simulink model "SimpleEKF_2007a"  (Simulink 6.6)
settings: Solver=FixedStepDiscrete  StartTime=0.0  StopTime=300  FixedStep=0.01  RelTol=1e-3
values from neighbouring files (symbols this model uses):
  initP = diag([ 1 1 1 1e5 1e5 1 1e5 1e5 1e5 ])    [SimpleEKF_init.m.m]
undefined symbols (not defined in the file or in its folder): DiscIntNeverNeededParam, gcbh, hwbcalib_subsystem
libraries: simulink x8, dspmtrx3 x5, dspinverses x1
(part 5 of 9)

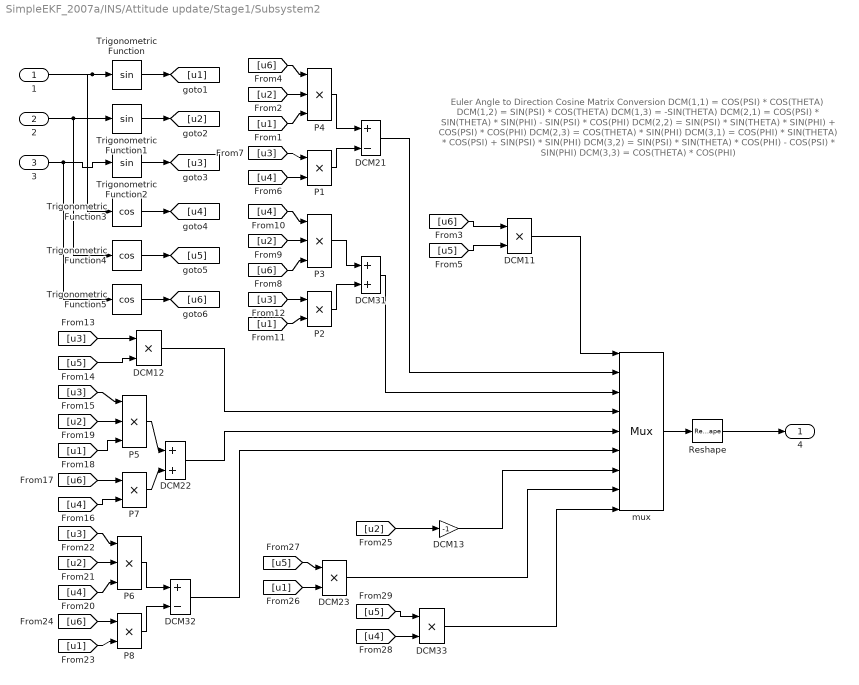
== system SimpleEKF_2007a/INS/Attitude update/Stage1/Subsystem2 ==
  note: Euler Angle to Direction Cosine Matrix Conversion
      |
      | DCM(1,1) = COS(PSI) * COS(THETA)
      | DCM(1,2) = SIN(PSI) * COS(THETA)
      | DCM(1,3) = -SIN(THETA)
      | DCM(2,1) = COS(PSI) * SIN(THETA) * SIN(PHI) - SIN(PSI) * COS(PHI)
      | DCM(2,2) = SIN(PSI) * SIN(THETA) * SIN(PHI) + COS(PSI) * COS(PHI)
      | DCM(2,3) = COS(THETA) * SIN(PHI)
      | DCM(3,1) = COS(PHI) * SIN(THETA) * COS(PSI) + SIN(PSI) * SIN(PHI)
      | DCM(3,2) = SIN(PSI) * SIN(THETA) * COS(PHI) - COS(PSI) * SIN(PHI)
      | DCM(3,3) = COS(THETA) * COS(PHI)
  1 : Inport  PortDimensions=1  DataType=double  OutDataType=fixdt(1,16,0)  OutScaling=[]
  2 : Inport  Port=2  PortDimensions=1  DataType=double  OutDataType=fixdt(1,16,0)  OutScaling=[]
  3 : Inport  Port=3  PortDimensions=1  DataType=double  OutDataType=fixdt(1,16,0)  OutScaling=[]
  DCM11 : Product  Tag=MBDLibrary v2007b.1  OutDataType=fixdt(1,16,0)  OutScaling=[]  RndMeth=Zero  InputSameDT=on  mask(Product (MBDLibrary)){Inputs_mbdlib=2}
      mask prompts: Inputs_mbdlib "Number of Inputs"
      mask help: Multiplies inputs.
      settings: OpenFcn=|
      | if exist('mbdlib_dialog')
      |    mbdlib_dialog(gcb,'open')
      | else
      |    open_system(gcb, 'mask')
      | end
      mask Help: The PRODUCT block is used to multiply inputs.
  DCM12 : Product  Tag=MBDLibrary v2007b.1  OutDataType=fixdt(1,16,0)  OutScaling=[]  RndMeth=Zero  InputSameDT=on  mask(Product (MBDLibrary)){Inputs_mbdlib=2}
      mask prompts: Inputs_mbdlib "Number of Inputs"
      mask help: Multiplies inputs.
      settings: OpenFcn=|
      | if exist('mbdlib_dialog')
      |    mbdlib_dialog(gcb,'open')
      | else
      |    open_system(gcb, 'mask')
      | end
      mask Help: The PRODUCT block is used to multiply inputs.
  DCM13 : Gain  Tag=MBDLibrary v2007b.1  Gain=-1  ParameterDataType=fixdt(1,16,0)  ParameterScaling=[]  OutDataType=fixdt(1,16,0)  OutScaling=[]  RndMeth=Zero  mask(Gain (MBDLibrary)){gain_mbdlib=-1}
      mask prompts: gain_mbdlib "Gain"
      mask help: Multiplies the input by the gain.
      settings: OpenFcn=|
      | if exist('mbdlib_dialog')
      |    mbdlib_dialog(gcb,'open')
      | else
      |    open_system(gcb, 'mask')
      | end
      mask Help: The GAIN block multiplies the input by the gain value.  This block may accept any data types other than boolean.  The user must take care to not use a non-integer gain for int32/uint32 inputs.
      mask Display: disp([get_param(gcb, 'Gain') 'x'])
  DCM21 : Sum  Tag=MBDLibrary v2007b.1  Inputs=+-  OutDataType=fixdt(1,16,0)  OutScaling=[]  RndMeth=Zero  InputSameDT=on  mask(Sum (MBDLibrary)){inputs_mbdlib=+-}
      mask prompts: inputs_mbdlib "List of signs"
      mask help: Adds values together.
      settings: OpenFcn=|
      | if exist('mbdlib_dialog')
      |    mbdlib_dialog(gcb,'open')
      | else
      |    open_system(gcb, 'mask')
      | end
      mask Help:
      | The SUM block is used to add or subtract  inputs.
      | The inputs may be specified as:
      |   (a) + or - for each port (i.e. ++-+)
      |   (b) An integer to indicate the number of ports to add
      | Note that the number of ports input to this block must be between 1 and 25.
      | When only 1 inport is selected, the block computes the summation of vector input elements and outputs a scalar.
  DCM22 : Sum  Tag=MBDLibrary v2007b.1  OutDataType=fixdt(1,16,0)  OutScaling=[]  RndMeth=Zero  InputSameDT=on  mask(Sum (MBDLibrary)){inputs_mbdlib=++}
      mask prompts: inputs_mbdlib "List of signs"
      mask help: Adds values together.
      settings: OpenFcn=|
      | if exist('mbdlib_dialog')
      |    mbdlib_dialog(gcb,'open')
      | else
      |    open_system(gcb, 'mask')
      | end
      mask Help:
      | The SUM block is used to add or subtract  inputs.
      | The inputs may be specified as:
      |   (a) + or - for each port (i.e. ++-+)
      |   (b) An integer to indicate the number of ports to add
      | Note that the number of ports input to this block must be between 1 and 25.
      | When only 1 inport is selected, the block computes the summation of vector input elements and outputs a scalar.
  DCM23 : Product  Tag=MBDLibrary v2007b.1  OutDataType=fixdt(1,16,0)  OutScaling=[]  RndMeth=Zero  InputSameDT=on  mask(Product (MBDLibrary)){Inputs_mbdlib=2}
      mask prompts: Inputs_mbdlib "Number of Inputs"
      mask help: Multiplies inputs.
      settings: OpenFcn=|
      | if exist('mbdlib_dialog')
      |    mbdlib_dialog(gcb,'open')
      | else
      |    open_system(gcb, 'mask')
      | end
      mask Help: The PRODUCT block is used to multiply inputs.
  DCM31 : Sum  Tag=MBDLibrary v2007b.1  OutDataType=fixdt(1,16,0)  OutScaling=[]  RndMeth=Zero  InputSameDT=on  mask(Sum (MBDLibrary)){inputs_mbdlib=++}
      mask prompts: inputs_mbdlib "List of signs"
      mask help: Adds values together.
      settings: OpenFcn=|
      | if exist('mbdlib_dialog')
      |    mbdlib_dialog(gcb,'open')
      | else
      |    open_system(gcb, 'mask')
      | end
      mask Help:
      | The SUM block is used to add or subtract  inputs.
      | The inputs may be specified as:
      |   (a) + or - for each port (i.e. ++-+)
      |   (b) An integer to indicate the number of ports to add
      | Note that the number of ports input to this block must be between 1 and 25.
      | When only 1 inport is selected, the block computes the summation of vector input elements and outputs a scalar.
  DCM32 : Sum  Tag=MBDLibrary v2007b.1  Inputs=+-  OutDataType=fixdt(1,16,0)  OutScaling=[]  RndMeth=Zero  InputSameDT=on  mask(Sum (MBDLibrary)){inputs_mbdlib=+-}
      mask prompts: inputs_mbdlib "List of signs"
      mask help: Adds values together.
      settings: OpenFcn=|
      | if exist('mbdlib_dialog')
      |    mbdlib_dialog(gcb,'open')
      | else
      |    open_system(gcb, 'mask')
      | end
      mask Help:
      | The SUM block is used to add or subtract  inputs.
      | The inputs may be specified as:
      |   (a) + or - for each port (i.e. ++-+)
      |   (b) An integer to indicate the number of ports to add
      | Note that the number of ports input to this block must be between 1 and 25.
      | When only 1 inport is selected, the block computes the summation of vector input elements and outputs a scalar.
  DCM33 : Product  Tag=MBDLibrary v2007b.1  OutDataType=fixdt(1,16,0)  OutScaling=[]  RndMeth=Zero  InputSameDT=on  mask(Product (MBDLibrary)){Inputs_mbdlib=2}
      mask prompts: Inputs_mbdlib "Number of Inputs"
      mask help: Multiplies inputs.
      settings: OpenFcn=|
      | if exist('mbdlib_dialog')
      |    mbdlib_dialog(gcb,'open')
      | else
      |    open_system(gcb, 'mask')
      | end
      mask Help: The PRODUCT block is used to multiply inputs.
  P1 : Product  Tag=MBDLibrary v2007b.1  OutDataType=fixdt(1,16,0)  OutScaling=[]  RndMeth=Zero  InputSameDT=on  mask(Product (MBDLibrary)){Inputs_mbdlib=2}
      mask prompts: Inputs_mbdlib "Number of Inputs"
      mask help: Multiplies inputs.
      settings: OpenFcn=|
      | if exist('mbdlib_dialog')
      |    mbdlib_dialog(gcb,'open')
      | else
      |    open_system(gcb, 'mask')
      | end
      mask Help: The PRODUCT block is used to multiply inputs.
  P2 : Product  Tag=MBDLibrary v2007b.1  OutDataType=fixdt(1,16,0)  OutScaling=[]  RndMeth=Zero  InputSameDT=on  mask(Product (MBDLibrary)){Inputs_mbdlib=2}
      mask prompts: Inputs_mbdlib "Number of Inputs"
      mask help: Multiplies inputs.
      settings: OpenFcn=|
      | if exist('mbdlib_dialog')
      |    mbdlib_dialog(gcb,'open')
      | else
      |    open_system(gcb, 'mask')
      | end
      mask Help: The PRODUCT block is used to multiply inputs.
  P3 : Product  Tag=MBDLibrary v2007b.1  Inputs=3  OutDataType=fixdt(1,16,0)  OutScaling=[]  RndMeth=Zero  InputSameDT=on  mask(Product (MBDLibrary)){Inputs_mbdlib=3}
      mask prompts: Inputs_mbdlib "Number of Inputs"
      mask help: Multiplies inputs.
      settings: OpenFcn=|
      | if exist('mbdlib_dialog')
      |    mbdlib_dialog(gcb,'open')
      | else
      |    open_system(gcb, 'mask')
      | end
      mask Help: The PRODUCT block is used to multiply inputs.
  P4 : Product  Tag=MBDLibrary v2007b.1  Inputs=3  OutDataType=fixdt(1,16,0)  OutScaling=[]  RndMeth=Zero  InputSameDT=on  mask(Product (MBDLibrary)){Inputs_mbdlib=3}
      mask prompts: Inputs_mbdlib "Number of Inputs"
      mask help: Multiplies inputs.
      settings: OpenFcn=|
      | if exist('mbdlib_dialog')
      |    mbdlib_dialog(gcb,'open')
      | else
      |    open_system(gcb, 'mask')
      | end
      mask Help: The PRODUCT block is used to multiply inputs.
  P5 : Product  Tag=MBDLibrary v2007b.1  Inputs=3  OutDataType=fixdt(1,16,0)  OutScaling=[]  RndMeth=Zero  InputSameDT=on  mask(Product (MBDLibrary)){Inputs_mbdlib=3}
      mask prompts: Inputs_mbdlib "Number of Inputs"
      mask help: Multiplies inputs.
      settings: OpenFcn=|
      | if exist('mbdlib_dialog')
      |    mbdlib_dialog(gcb,'open')
      | else
      |    open_system(gcb, 'mask')
      | end
      mask Help: The PRODUCT block is used to multiply inputs.
  P6 : Product  Tag=MBDLibrary v2007b.1  Inputs=3  OutDataType=fixdt(1,16,0)  OutScaling=[]  RndMeth=Zero  InputSameDT=on  mask(Product (MBDLibrary)){Inputs_mbdlib=3}
      mask prompts: Inputs_mbdlib "Number of Inputs"
      mask help: Multiplies inputs.
      settings: OpenFcn=|
      | if exist('mbdlib_dialog')
      |    mbdlib_dialog(gcb,'open')
      | else
      |    open_system(gcb, 'mask')
      | end
      mask Help: The PRODUCT block is used to multiply inputs.
  P7 : Product  Tag=MBDLibrary v2007b.1  OutDataType=fixdt(1,16,0)  OutScaling=[]  RndMeth=Zero  InputSameDT=on  mask(Product (MBDLibrary)){Inputs_mbdlib=2}
      mask prompts: Inputs_mbdlib "Number of Inputs"
      mask help: Multiplies inputs.
      settings: OpenFcn=|
      | if exist('mbdlib_dialog')
      |    mbdlib_dialog(gcb,'open')
      | else
      |    open_system(gcb, 'mask')
      | end
      mask Help: The PRODUCT block is used to multiply inputs.
  P8 : Product  Tag=MBDLibrary v2007b.1  OutDataType=fixdt(1,16,0)  OutScaling=[]  RndMeth=Zero  InputSameDT=on  mask(Product (MBDLibrary)){Inputs_mbdlib=2}
      mask prompts: Inputs_mbdlib "Number of Inputs"
      mask help: Multiplies inputs.
      settings: OpenFcn=|
      | if exist('mbdlib_dialog')
      |    mbdlib_dialog(gcb,'open')
      | else
      |    open_system(gcb, 'mask')
      | end
      mask Help: The PRODUCT block is used to multiply inputs.
  Reshape : Reshape  OutputDimensionality=Customize  OutputDimensions=[3,3]
  Trigonometric Function : Trigonometry
  Trigonometric Function1 : Trigonometry
  Trigonometric Function2 : Trigonometry
  Trigonometric Function3 : Trigonometry  Operator=cos
  Trigonometric Function4 : Trigonometry  Operator=cos
  Trigonometric Function5 : Trigonometry  Operator=cos
  mux : Mux  Tag=MBDLibrary v2007b.1  Inputs=9  mask(Mux (MBDLibrary)){Inputs_mbdlib=9}
      mask prompts: Inputs_mbdlib "Number of Inputs"
      mask help: Converts multipule inputs to a vector.
      settings: OpenFcn=|
      | if exist('mbdlib_dialog')
      |    mbdlib_dialog(gcb,'open')
      | else
      |    open_system(gcb, 'mask')
      | end
      mask Help: The MUX block provides a vector output to the model for separate inputs.  The output order will correspond to the input order (from the first input at the top of the block to the last input at the bottom of the block).
  4 : Outport  OutDataType=fixdt(1,16,0)  OutScaling=[]  InitialOutput=0
  wires:
  [u6] -> P3/3
  [u2] -> P3/2
  [u4] -> P3/1
  mux/1 -> Reshape/1
  DCM12/1 -> mux/4
  Reshape/1 -> 4/1
  1/1 -> Trigonometric Function/1, Trigonometric Function3/1
  2/1 -> Trigonometric Function1/1, Trigonometric Function4/1
  3/1 -> Trigonometric Function2/1, Trigonometric Function5/1
  Trigonometric Function/1 -> [u1]
  Trigonometric Function1/1 -> [u2]
  Trigonometric Function2/1 -> [u3]
  Trigonometric Function3/1 -> [u4]
  Trigonometric Function4/1 -> [u5]
  Trigonometric Function5/1 -> [u6]
  [u6] -> P4/1
  [u2] -> P4/2
  [u1] -> P4/3
  [u3] -> P1/1
  [u4] -> P1/2
  P4/1 -> DCM21/1
  P1/1 -> DCM21/2
  [u3] -> P2/1
  [u1] -> P2/2
  P3/1 -> DCM31/1
  P2/1 -> DCM31/2
  DCM21/1 -> mux/2
  DCM31/1 -> mux/3
  [u3] -> DCM12/1
  [u5] -> DCM12/2
  [u3] -> P5/1
  [u2] -> P5/2
  [u1] -> P5/3
  [u6] -> P7/1
  [u4] -> P7/2
  P5/1 -> DCM22/1
  P7/1 -> DCM22/2
  DCM22/1 -> mux/5
  [u3] -> P6/1
  [u2] -> P6/2
  [u4] -> P6/3
  [u6] -> P8/1
  [u1] -> P8/2
  P6/1 -> DCM32/1
  P8/1 -> DCM32/2
  DCM32/1 -> mux/6
  [u6] -> DCM11/1
  [u5] -> DCM11/2
  DCM11/1 -> mux/1
  [u2] -> DCM13/1
  DCM13/1 -> mux/7
  [u1] -> DCM23/2
  [u5] -> DCM23/1
  DCM23/1 -> mux/8
  [u4] -> DCM33/2
  [u5] -> DCM33/1
  DCM33/1 -> mux/9

== system SimpleEKF_2007a/INS/Attitude update/Stage1/square ==
  squareLibIn : Inport  DataType=double  OutDataType=fixdt(1,16,0)  OutScaling=[]
  Product : Product  OutDataType=fixdt(1,16,0)  OutScaling=[]  RndMeth=Zero
  squareLibOut : Outport  OutDataType=fixdt(1,16,0)  OutScaling=[]  InitialOutput=0
  wires:
  squareLibIn/1 -> Product/2, Product/1
  Product/1 -> squareLibOut/1

== system SimpleEKF_2007a/INS/Attitude update/Stage1/square1 ==
  squareLibIn : Inport  DataType=double  OutDataType=fixdt(1,16,0)  OutScaling=[]
  Product : Product  OutDataType=fixdt(1,16,0)  OutScaling=[]  RndMeth=Zero
  squareLibOut : Outport  OutDataType=fixdt(1,16,0)  OutScaling=[]  InitialOutput=0
  wires:
  squareLibIn/1 -> Product/2, Product/1
  Product/1 -> squareLibOut/1

== system SimpleEKF_2007a/INS/Attitude update/Stage1/square2 ==
  squareLibIn : Inport  DataType=double  OutDataType=fixdt(1,16,0)  OutScaling=[]
  Product : Product  OutDataType=fixdt(1,16,0)  OutScaling=[]  RndMeth=Zero
  squareLibOut : Outport  OutDataType=fixdt(1,16,0)  OutScaling=[]  InitialOutput=0
  wires:
  squareLibIn/1 -> Product/2, Product/1
  Product/1 -> squareLibOut/1

== system SimpleEKF_2007a/INS/Attitude update/Stage2/Subsystem ==
  Quat : Inport  PortDimensions=4  OutDataType=fixdt(1,16,0)  OutScaling=[]
  Subsystem : Subsystem
  a11 : Subsystem  InitFcn=%hwbcalib_subsystem(gcbh,99);
      settings: AttributesFormatString=(Page 13)  CopyFcn=hwbcalib_copyfcn(gcbh);  DeleteFcn=hwbcalib_subsystem(gcbh,'delete');
      mask Type: Subsystem (HW)
      mask Display:
      | port_label('input',1,'quat');
      | port_label('output',1,'a11');
  a12 : Subsystem  InitFcn=%hwbcalib_subsystem(gcbh,99);
      settings: AttributesFormatString=(Page 14)  CopyFcn=hwbcalib_copyfcn(gcbh);  DeleteFcn=hwbcalib_subsystem(gcbh,'delete');
      mask Type: Subsystem (HW)
      mask Display:
      | port_label('input',1,'quat');
      | port_label('output',1,'a12');
  a13 : Subsystem  InitFcn=%hwbcalib_subsystem(gcbh,99);
      settings: AttributesFormatString=(Page 15)  CopyFcn=hwbcalib_copyfcn(gcbh);  DeleteFcn=hwbcalib_subsystem(gcbh,'delete');
      mask Type: Subsystem (HW)
      mask Display:
      | port_label('input',1,'quat');
      | port_label('output',1,'a13');
  a21 : Subsystem  InitFcn=%hwbcalib_subsystem(gcbh,99);
      settings: AttributesFormatString=(Page 16)  CopyFcn=hwbcalib_copyfcn(gcbh);  DeleteFcn=hwbcalib_subsystem(gcbh,'delete');
      mask Type: Subsystem (HW)
      mask Display:
      | port_label('input',1,'quat');
      | port_label('output',1,'a21');
  a22 : Subsystem  InitFcn=%hwbcalib_subsystem(gcbh,99);
      settings: AttributesFormatString=(Page 17)  CopyFcn=hwbcalib_copyfcn(gcbh);  DeleteFcn=hwbcalib_subsystem(gcbh,'delete');
      mask Type: Subsystem (HW)
      mask Display:
      | port_label('input',1,'quat');
      | port_label('output',1,'a22');
  a23 : Subsystem  InitFcn=%hwbcalib_subsystem(gcbh,99);
      settings: AttributesFormatString=(Page 18)  CopyFcn=hwbcalib_copyfcn(gcbh);  DeleteFcn=hwbcalib_subsystem(gcbh,'delete');
      mask Type: Subsystem (HW)
      mask Display:
      | port_label('input',1,'quat');
      | port_label('output',1,'a23');
  a31 : Subsystem  InitFcn=%hwbcalib_subsystem(gcbh,99);
      settings: AttributesFormatString=(Page 19)  CopyFcn=hwbcalib_copyfcn(gcbh);  DeleteFcn=hwbcalib_subsystem(gcbh,'delete');
      mask Type: Subsystem (HW)
      mask Display:
      | port_label('input',1,'quat');
      | port_label('output',1,'a31');
  a32 : Subsystem  InitFcn=%hwbcalib_subsystem(gcbh,99);
      settings: AttributesFormatString=(Page 20)  CopyFcn=hwbcalib_copyfcn(gcbh);  DeleteFcn=hwbcalib_subsystem(gcbh,'delete');
      mask Type: Subsystem (HW)
      mask Display:
      | port_label('input',1,'quat');
      | port_label('output',1,'a32');
  a33 : Subsystem  InitFcn=%hwbcalib_subsystem(gcbh,99);
      settings: AttributesFormatString=(Page 21)  CopyFcn=hwbcalib_copyfcn(gcbh);  DeleteFcn=hwbcalib_subsystem(gcbh,'delete');
      mask Type: Subsystem (HW)
      mask Display:
      | port_label('input',1,'quat');
      | port_label('output',1,'a33');
  quat normalize : Subsystem
  DCM : Outport  PortDimensions=[3,3]  OutDataType=fixdt(1,16,0)  OutScaling=[]  InitialOutput=0
  wires:
  Quat/1 -> quat normalize/1(q)
  Subsystem/1(Matrix) -> DCM/1
  quat normalize/1(normal(q)) -> a11/1(quat), a21/1(quat), a31/1(quat), a12/1(quat), a22/1(quat), a32/1(quat), a13/1(quat), a23/1(quat), a33/1(quat)
  a11/1(a11) -> Subsystem/1(M11)
  a21/1(a21) -> Subsystem/2(M21)
  a31/1(a31) -> Subsystem/3(M31)
  a12/1(a12) -> Subsystem/4(M12)
  a22/1(a22) -> Subsystem/5(M22)
  a32/1(a32) -> Subsystem/6(M32)
  a13/1(a13) -> Subsystem/7(M13)
  a23/1(a23) -> Subsystem/8(M23)
  a33/1(a33) -> Subsystem/9(M33)

== system SimpleEKF_2007a/INS/Attitude update/Stage2/Subsystem1 ==
  note: Direction Cosine Matrix to Euler Angle Conversion
      |
      | Roll = ATAN2(SIN(PHI)*COS(THETA),COS(PHI)*COS(THETA))
      | Pitch = ASIN(SIN(THETA))
      | Yaw = ATAN2(SIN(PSI)*COS(THETA),COS(PSI)*COS(THETA))
  1 : Inport  PortDimensions=[3 3]  DataType=double  OutDataType=fixdt(1,16,0)  OutScaling=[]
  Reshape : Reshape  OutputDimensionality=Customize  OutputDimensions=[9,1]
  Trigonometric Function : Trigonometry  Operator=asin
  Trigonometric Function1 : Trigonometry  Operator=atan2
  Trigonometric Function2 : Trigonometry  Operator=atan2
  gain : Gain  Tag=MBDLibrary v2007b.1  Gain=-1  ParameterDataType=fixdt(1,16,0)  ParameterScaling=[]  OutDataType=fixdt(1,16,0)  OutScaling=[]  RndMeth=Zero  mask(Gain (MBDLibrary)){gain_mbdlib=-1}
      mask prompts: gain_mbdlib "Gain"
      mask help: Multiplies the input by the gain.
      settings: OpenFcn=|
      | if exist('mbdlib_dialog')
      |    mbdlib_dialog(gcb,'open')
      | else
      |    open_system(gcb, 'mask')
      | end
      mask Help: The GAIN block multiplies the input by the gain value.  This block may accept any data types other than boolean.  The user must take care to not use a non-integer gain for int32/uint32 inputs.
      mask Display: disp([get_param(gcb, 'Gain') 'x'])
  limit : Saturate  Tag=MBDLibrary v2007b.1  UpperLimit=1  LowerLimit=-1  ZeroCross=off  mask(Limit (MBDLibrary)){UpperLimit_mbdlib=1, LowerLimit_mbdlib=-1}
      mask prompts: UpperLimit_mbdlib "Upper Limit"; LowerLimit_mbdlib "Lower Limit"
      mask help: Provides upper and lower bounds for a signal.
      settings: AttributesFormatString={%<LowerLimit> to %<UpperLimit>}
      settings: OpenFcn=|
      | if exist('mbdlib_dialog')
      |    mbdlib_dialog(gcb,'open')
      | else
      |    open_system(gcb, 'mask')
      | end
      mask Help: The  LIMITER block provides upper and lower bounds for a signal.  If the input is between the boundaries, it is passed directly to the output.  If the input is greater than the upper bound, it will be output as the upper boundary value.  If the input is less than the lower bound, it will be output as the lower boundary value.  This block will accept any except Boolean inputs, and is vectorized.
  selector : Selector  Tag=MBDLibrary v2007b.1  IndexOptions=Index vector (dialog)  Indices=8  OutputSizes=1  InputPortWidth=9  mask(Mux Selector (MBDLibrary)){InputPortWidth_mbdlib=9, Indices_mbdlib=8}
      mask prompts: InputPortWidth_mbdlib "Input Port Width"; Indices_mbdlib "Output Indices"
      mask help: Changes the order of the inputs.
      settings: OpenFcn=|
      | if exist('mbdlib_dialog')
      |    mbdlib_dialog(gcb,'open')
      | else
      |    open_system(gcb, 'mask')
      | end
      settings: CloseFcn=|
      | if exist('mbdlib_selector')
      |    mbdlib_selector(gcb)
      | end
      mask Help: The SELECTOR block is a MULTIPLEXED SELECTOR block, used to change the input/output order of a multiplexed data stream.
      mask Display:
      | port_label('input', 1,'[9]')
      | text(1.0,0.5,'8', 'horizontalAlignment', 'right')
  selector1 : Selector  Tag=MBDLibrary v2007b.1  IndexOptions=Index vector (dialog)  Indices=9  OutputSizes=1  InputPortWidth=9  mask(Mux Selector (MBDLibrary)){InputPortWidth_mbdlib=9, Indices_mbdlib=9}
      mask prompts: InputPortWidth_mbdlib "Input Port Width"; Indices_mbdlib "Output Indices"
      mask help: Changes the order of the inputs.
      settings: OpenFcn=|
      | if exist('mbdlib_dialog')
      |    mbdlib_dialog(gcb,'open')
      | else
      |    open_system(gcb, 'mask')
      | end
      settings: CloseFcn=|
      | if exist('mbdlib_selector')
      |    mbdlib_selector(gcb)
      | end
      mask Help: The SELECTOR block is a MULTIPLEXED SELECTOR block, used to change the input/output order of a multiplexed data stream.
      mask Display:
      | port_label('input', 1,'[9]')
      | text(1.0,0.5,'9', 'horizontalAlignment', 'right')
  selector2 : Selector  Tag=MBDLibrary v2007b.1  IndexOptions=Index vector (dialog)  Indices=7  OutputSizes=1  InputPortWidth=9  mask(Mux Selector (MBDLibrary)){InputPortWidth_mbdlib=9, Indices_mbdlib=7}
      mask prompts: InputPortWidth_mbdlib "Input Port Width"; Indices_mbdlib "Output Indices"
      mask help: Changes the order of the inputs.
      settings: OpenFcn=|
      | if exist('mbdlib_dialog')
      |    mbdlib_dialog(gcb,'open')
      | else
      |    open_system(gcb, 'mask')
      | end
      settings: CloseFcn=|
      | if exist('mbdlib_selector')
      |    mbdlib_selector(gcb)
      | end
      mask Help: The SELECTOR block is a MULTIPLEXED SELECTOR block, used to change the input/output order of a multiplexed data stream.
      mask Display:
      | port_label('input', 1,'[9]')
      | text(1.0,0.5,'7', 'horizontalAlignment', 'right')
  selector3 : Selector  Tag=MBDLibrary v2007b.1  IndexOptions=Index vector (dialog)  Indices=4  OutputSizes=1  InputPortWidth=9  mask(Mux Selector (MBDLibrary)){InputPortWidth_mbdlib=9, Indices_mbdlib=4}
      mask prompts: InputPortWidth_mbdlib "Input Port Width"; Indices_mbdlib "Output Indices"
      mask help: Changes the order of the inputs.
      settings: OpenFcn=|
      | if exist('mbdlib_dialog')
      |    mbdlib_dialog(gcb,'open')
      | else
      |    open_system(gcb, 'mask')
      | end
      settings: CloseFcn=|
      | if exist('mbdlib_selector')
      |    mbdlib_selector(gcb)
      | end
      mask Help: The SELECTOR block is a MULTIPLEXED SELECTOR block, used to change the input/output order of a multiplexed data stream.
      mask Display:
      | port_label('input', 1,'[9]')
      | text(1.0,0.5,'4', 'horizontalAlignment', 'right')
  selector4 : Selector  Tag=MBDLibrary v2007b.1  IndexOptions=Index vector (dialog)  Indices=1  OutputSizes=1  InputPortWidth=9  mask(Mux Selector (MBDLibrary)){InputPortWidth_mbdlib=9, Indices_mbdlib=1}
      mask prompts: InputPortWidth_mbdlib "Input Port Width"; Indices_mbdlib "Output Indices"
      mask help: Changes the order of the inputs.
      settings: OpenFcn=|
      | if exist('mbdlib_dialog')
      |    mbdlib_dialog(gcb,'open')
      | else
      |    open_system(gcb, 'mask')
      | end
      settings: CloseFcn=|
      | if exist('mbdlib_selector')
      |    mbdlib_selector(gcb)
      | end
      mask Help: The SELECTOR block is a MULTIPLEXED SELECTOR block, used to change the input/output order of a multiplexed data stream.
      mask Display:
      | port_label('input', 1,'[9]')
      | text(1.0,0.5,'1', 'horizontalAlignment', 'right')
  2 : Outport  OutDataType=fixdt(1,16,0)  OutScaling=[]  InitialOutput=0
  3 : Outport  Port=2  OutDataType=fixdt(1,16,0)  OutScaling=[]  InitialOutput=0
  4 : Outport  Port=3  OutDataType=fixdt(1,16,0)  OutScaling=[]  InitialOutput=0
  wires:
  gain/1 -> selector2/1
  limit/1 -> Trigonometric Function/1
  1/1 -> Reshape/1
  Reshape/1 -> gain/1, selector1/1, selector/1, selector4/1, selector3/1
  selector2/1 -> limit/1
  selector/1 -> Trigonometric Function1/1
  selector1/1 -> Trigonometric Function1/2
  selector3/1 -> Trigonometric Function2/1
  selector4/1 -> Trigonometric Function2/2
  Trigonometric Function1/1 -> 2/1
  Trigonometric Function/1 -> 3/1
  Trigonometric Function2/1 -> 4/1

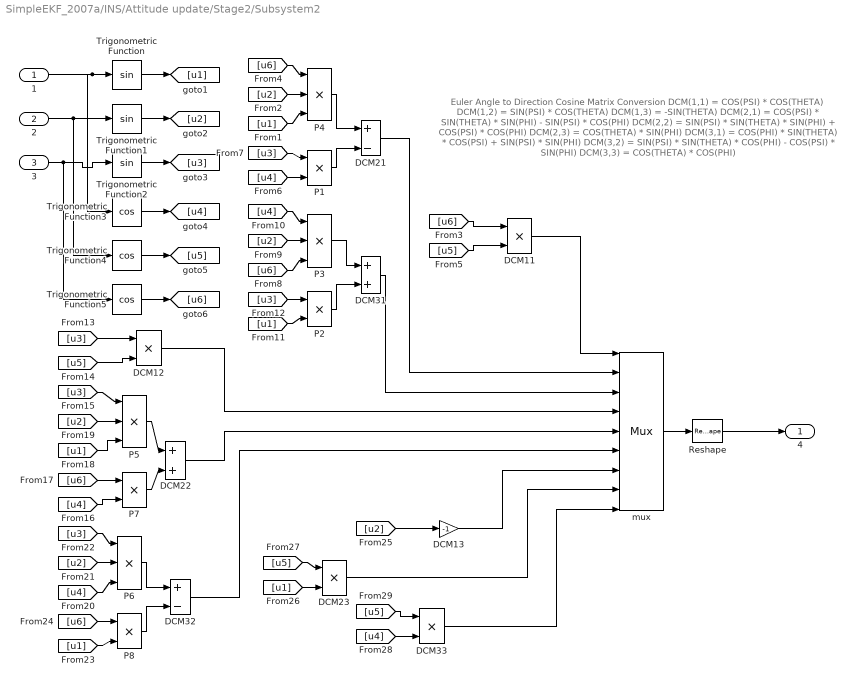
== system SimpleEKF_2007a/INS/Attitude update/Stage2/Subsystem2 ==
  note: Euler Angle to Direction Cosine Matrix Conversion
      |
      | DCM(1,1) = COS(PSI) * COS(THETA)
      | DCM(1,2) = SIN(PSI) * COS(THETA)
      | DCM(1,3) = -SIN(THETA)
      | DCM(2,1) = COS(PSI) * SIN(THETA) * SIN(PHI) - SIN(PSI) * COS(PHI)
      | DCM(2,2) = SIN(PSI) * SIN(THETA) * SIN(PHI) + COS(PSI) * COS(PHI)
      | DCM(2,3) = COS(THETA) * SIN(PHI)
      | DCM(3,1) = COS(PHI) * SIN(THETA) * COS(PSI) + SIN(PSI) * SIN(PHI)
      | DCM(3,2) = SIN(PSI) * SIN(THETA) * COS(PHI) - COS(PSI) * SIN(PHI)
      | DCM(3,3) = COS(THETA) * COS(PHI)
  1 : Inport  PortDimensions=1  DataType=double  OutDataType=fixdt(1,16,0)  OutScaling=[]
  2 : Inport  Port=2  PortDimensions=1  DataType=double  OutDataType=fixdt(1,16,0)  OutScaling=[]
  3 : Inport  Port=3  PortDimensions=1  DataType=double  OutDataType=fixdt(1,16,0)  OutScaling=[]
  DCM11 : Product  Tag=MBDLibrary v2007b.1  OutDataType=fixdt(1,16,0)  OutScaling=[]  RndMeth=Zero  InputSameDT=on  mask(Product (MBDLibrary)){Inputs_mbdlib=2}
      mask prompts: Inputs_mbdlib "Number of Inputs"
      mask help: Multiplies inputs.
      settings: OpenFcn=|
      | if exist('mbdlib_dialog')
      |    mbdlib_dialog(gcb,'open')
      | else
      |    open_system(gcb, 'mask')
      | end
      mask Help: The PRODUCT block is used to multiply inputs.
  DCM12 : Product  Tag=MBDLibrary v2007b.1  OutDataType=fixdt(1,16,0)  OutScaling=[]  RndMeth=Zero  InputSameDT=on  mask(Product (MBDLibrary)){Inputs_mbdlib=2}
      mask prompts: Inputs_mbdlib "Number of Inputs"
      mask help: Multiplies inputs.
      settings: OpenFcn=|
      | if exist('mbdlib_dialog')
      |    mbdlib_dialog(gcb,'open')
      | else
      |    open_system(gcb, 'mask')
      | end
      mask Help: The PRODUCT block is used to multiply inputs.
  DCM13 : Gain  Tag=MBDLibrary v2007b.1  Gain=-1  ParameterDataType=fixdt(1,16,0)  ParameterScaling=[]  OutDataType=fixdt(1,16,0)  OutScaling=[]  RndMeth=Zero  mask(Gain (MBDLibrary)){gain_mbdlib=-1}
      mask prompts: gain_mbdlib "Gain"
      mask help: Multiplies the input by the gain.
      settings: OpenFcn=|
      | if exist('mbdlib_dialog')
      |    mbdlib_dialog(gcb,'open')
      | else
      |    open_system(gcb, 'mask')
      | end
      mask Help: The GAIN block multiplies the input by the gain value.  This block may accept any data types other than boolean.  The user must take care to not use a non-integer gain for int32/uint32 inputs.
      mask Display: disp([get_param(gcb, 'Gain') 'x'])
  DCM21 : Sum  Tag=MBDLibrary v2007b.1  Inputs=+-  OutDataType=fixdt(1,16,0)  OutScaling=[]  RndMeth=Zero  InputSameDT=on  mask(Sum (MBDLibrary)){inputs_mbdlib=+-}
      mask prompts: inputs_mbdlib "List of signs"
      mask help: Adds values together.
      settings: OpenFcn=|
      | if exist('mbdlib_dialog')
      |    mbdlib_dialog(gcb,'open')
      | else
      |    open_system(gcb, 'mask')
      | end
      mask Help:
      | The SUM block is used to add or subtract  inputs.
      | The inputs may be specified as:
      |   (a) + or - for each port (i.e. ++-+)
      |   (b) An integer to indicate the number of ports to add
      | Note that the number of ports input to this block must be between 1 and 25.
      | When only 1 inport is selected, the block computes the summation of vector input elements and outputs a scalar.
  DCM22 : Sum  Tag=MBDLibrary v2007b.1  OutDataType=fixdt(1,16,0)  OutScaling=[]  RndMeth=Zero  InputSameDT=on  mask(Sum (MBDLibrary)){inputs_mbdlib=++}
      mask prompts: inputs_mbdlib "List of signs"
      mask help: Adds values together.
      settings: OpenFcn=|
      | if exist('mbdlib_dialog')
      |    mbdlib_dialog(gcb,'open')
      | else
      |    open_system(gcb, 'mask')
      | end
      mask Help:
      | The SUM block is used to add or subtract  inputs.
      | The inputs may be specified as:
      |   (a) + or - for each port (i.e. ++-+)
      |   (b) An integer to indicate the number of ports to add
      | Note that the number of ports input to this block must be between 1 and 25.
      | When only 1 inport is selected, the block computes the summation of vector input elements and outputs a scalar.
  DCM23 : Product  Tag=MBDLibrary v2007b.1  OutDataType=fixdt(1,16,0)  OutScaling=[]  RndMeth=Zero  InputSameDT=on  mask(Product (MBDLibrary)){Inputs_mbdlib=2}
      mask prompts: Inputs_mbdlib "Number of Inputs"
      mask help: Multiplies inputs.
      settings: OpenFcn=|
      | if exist('mbdlib_dialog')
      |    mbdlib_dialog(gcb,'open')
      | else
      |    open_system(gcb, 'mask')
      | end
      mask Help: The PRODUCT block is used to multiply inputs.
  DCM31 : Sum  Tag=MBDLibrary v2007b.1  OutDataType=fixdt(1,16,0)  OutScaling=[]  RndMeth=Zero  InputSameDT=on  mask(Sum (MBDLibrary)){inputs_mbdlib=++}
      mask prompts: inputs_mbdlib "List of signs"
      mask help: Adds values together.
      settings: OpenFcn=|
      | if exist('mbdlib_dialog')
      |    mbdlib_dialog(gcb,'open')
      | else
      |    open_system(gcb, 'mask')
      | end
      mask Help:
      | The SUM block is used to add or subtract  inputs.
      | The inputs may be specified as:
      |   (a) + or - for each port (i.e. ++-+)
      |   (b) An integer to indicate the number of ports to add
      | Note that the number of ports input to this block must be between 1 and 25.
      | When only 1 inport is selected, the block computes the summation of vector input elements and outputs a scalar.
  DCM32 : Sum  Tag=MBDLibrary v2007b.1  Inputs=+-  OutDataType=fixdt(1,16,0)  OutScaling=[]  RndMeth=Zero  InputSameDT=on  mask(Sum (MBDLibrary)){inputs_mbdlib=+-}
      mask prompts: inputs_mbdlib "List of signs"
      mask help: Adds values together.
      settings: OpenFcn=|
      | if exist('mbdlib_dialog')
      |    mbdlib_dialog(gcb,'open')
      | else
      |    open_system(gcb, 'mask')
      | end
      mask Help:
      | The SUM block is used to add or subtract  inputs.
      | The inputs may be specified as:
      |   (a) + or - for each port (i.e. ++-+)
      |   (b) An integer to indicate the number of ports to add
      | Note that the number of ports input to this block must be between 1 and 25.
      | When only 1 inport is selected, the block computes the summation of vector input elements and outputs a scalar.
  DCM33 : Product  Tag=MBDLibrary v2007b.1  OutDataType=fixdt(1,16,0)  OutScaling=[]  RndMeth=Zero  InputSameDT=on  mask(Product (MBDLibrary)){Inputs_mbdlib=2}
      mask prompts: Inputs_mbdlib "Number of Inputs"
      mask help: Multiplies inputs.
      settings: OpenFcn=|
      | if exist('mbdlib_dialog')
      |    mbdlib_dialog(gcb,'open')
      | else
      |    open_system(gcb, 'mask')
      | end
      mask Help: The PRODUCT block is used to multiply inputs.
  P1 : Product  Tag=MBDLibrary v2007b.1  OutDataType=fixdt(1,16,0)  OutScaling=[]  RndMeth=Zero  InputSameDT=on  mask(Product (MBDLibrary)){Inputs_mbdlib=2}
      mask prompts: Inputs_mbdlib "Number of Inputs"
      mask help: Multiplies inputs.
      settings: OpenFcn=|
      | if exist('mbdlib_dialog')
      |    mbdlib_dialog(gcb,'open')
      | else
      |    open_system(gcb, 'mask')
      | end
      mask Help: The PRODUCT block is used to multiply inputs.
  P2 : Product  Tag=MBDLibrary v2007b.1  OutDataType=fixdt(1,16,0)  OutScaling=[]  RndMeth=Zero  InputSameDT=on  mask(Product (MBDLibrary)){Inputs_mbdlib=2}
      mask prompts: Inputs_mbdlib "Number of Inputs"
      mask help: Multiplies inputs.
      settings: OpenFcn=|
      | if exist('mbdlib_dialog')
      |    mbdlib_dialog(gcb,'open')
      | else
      |    open_system(gcb, 'mask')
      | end
      mask Help: The PRODUCT block is used to multiply inputs.
  P3 : Product  Tag=MBDLibrary v2007b.1  Inputs=3  OutDataType=fixdt(1,16,0)  OutScaling=[]  RndMeth=Zero  InputSameDT=on  mask(Product (MBDLibrary)){Inputs_mbdlib=3}
      mask prompts: Inputs_mbdlib "Number of Inputs"
      mask help: Multiplies inputs.
      settings: OpenFcn=|
      | if exist('mbdlib_dialog')
      |    mbdlib_dialog(gcb,'open')
      | else
      |    open_system(gcb, 'mask')
      | end
      mask Help: The PRODUCT block is used to multiply inputs.
  P4 : Product  Tag=MBDLibrary v2007b.1  Inputs=3  OutDataType=fixdt(1,16,0)  OutScaling=[]  RndMeth=Zero  InputSameDT=on  mask(Product (MBDLibrary)){Inputs_mbdlib=3}
      mask prompts: Inputs_mbdlib "Number of Inputs"
      mask help: Multiplies inputs.
      settings: OpenFcn=|
      | if exist('mbdlib_dialog')
      |    mbdlib_dialog(gcb,'open')
      | else
      |    open_system(gcb, 'mask')
      | end
      mask Help: The PRODUCT block is used to multiply inputs.
  P5 : Product  Tag=MBDLibrary v2007b.1  Inputs=3  OutDataType=fixdt(1,16,0)  OutScaling=[]  RndMeth=Zero  InputSameDT=on  mask(Product (MBDLibrary)){Inputs_mbdlib=3}
      mask prompts: Inputs_mbdlib "Number of Inputs"
      mask help: Multiplies inputs.
      settings: OpenFcn=|
      | if exist('mbdlib_dialog')
      |    mbdlib_dialog(gcb,'open')
      | else
      |    open_system(gcb, 'mask')
      | end
      mask Help: The PRODUCT block is used to multiply inputs.
  P6 : Product  Tag=MBDLibrary v2007b.1  Inputs=3  OutDataType=fixdt(1,16,0)  OutScaling=[]  RndMeth=Zero  InputSameDT=on  mask(Product (MBDLibrary)){Inputs_mbdlib=3}
      mask prompts: Inputs_mbdlib "Number of Inputs"
      mask help: Multiplies inputs.
      settings: OpenFcn=|
      | if exist('mbdlib_dialog')
      |    mbdlib_dialog(gcb,'open')
      | else
      |    open_system(gcb, 'mask')
      | end
      mask Help: The PRODUCT block is used to multiply inputs.
  P7 : Product  Tag=MBDLibrary v2007b.1  OutDataType=fixdt(1,16,0)  OutScaling=[]  RndMeth=Zero  InputSameDT=on  mask(Product (MBDLibrary)){Inputs_mbdlib=2}
      mask prompts: Inputs_mbdlib "Number of Inputs"
      mask help: Multiplies inputs.
      settings: OpenFcn=|
      | if exist('mbdlib_dialog')
      |    mbdlib_dialog(gcb,'open')
      | else
      |    open_system(gcb, 'mask')
      | end
      mask Help: The PRODUCT block is used to multiply inputs.
  P8 : Product  Tag=MBDLibrary v2007b.1  OutDataType=fixdt(1,16,0)  OutScaling=[]  RndMeth=Zero  InputSameDT=on  mask(Product (MBDLibrary)){Inputs_mbdlib=2}
      mask prompts: Inputs_mbdlib "Number of Inputs"
      mask help: Multiplies inputs.
      settings: OpenFcn=|
      | if exist('mbdlib_dialog')
      |    mbdlib_dialog(gcb,'open')
      | else
      |    open_system(gcb, 'mask')
      | end
      mask Help: The PRODUCT block is used to multiply inputs.
  Reshape : Reshape  OutputDimensionality=Customize  OutputDimensions=[3,3]
  Trigonometric Function : Trigonometry
  Trigonometric Function1 : Trigonometry
  Trigonometric Function2 : Trigonometry
  Trigonometric Function3 : Trigonometry  Operator=cos
  Trigonometric Function4 : Trigonometry  Operator=cos
  Trigonometric Function5 : Trigonometry  Operator=cos
  mux : Mux  Tag=MBDLibrary v2007b.1  Inputs=9  mask(Mux (MBDLibrary)){Inputs_mbdlib=9}
      mask prompts: Inputs_mbdlib "Number of Inputs"
      mask help: Converts multipule inputs to a vector.
      settings: OpenFcn=|
      | if exist('mbdlib_dialog')
      |    mbdlib_dialog(gcb,'open')
      | else
      |    open_system(gcb, 'mask')
      | end
      mask Help: The MUX block provides a vector output to the model for separate inputs.  The output order will correspond to the input order (from the first input at the top of the block to the last input at the bottom of the block).
  4 : Outport  OutDataType=fixdt(1,16,0)  OutScaling=[]  InitialOutput=0
  wires:
  [u6] -> P3/3
  [u2] -> P3/2
  [u4] -> P3/1
  mux/1 -> Reshape/1
  DCM12/1 -> mux/4
  Reshape/1 -> 4/1
  1/1 -> Trigonometric Function/1, Trigonometric Function3/1
  2/1 -> Trigonometric Function1/1, Trigonometric Function4/1
  3/1 -> Trigonometric Function2/1, Trigonometric Function5/1
  Trigonometric Function/1 -> [u1]
  Trigonometric Function1/1 -> [u2]
  Trigonometric Function2/1 -> [u3]
  Trigonometric Function3/1 -> [u4]
  Trigonometric Function4/1 -> [u5]
  Trigonometric Function5/1 -> [u6]
  [u6] -> P4/1
  [u2] -> P4/2
  [u1] -> P4/3
  [u3] -> P1/1
  [u4] -> P1/2
  P4/1 -> DCM21/1
  P1/1 -> DCM21/2
  [u3] -> P2/1
  [u1] -> P2/2
  P3/1 -> DCM31/1
  P2/1 -> DCM31/2
  DCM21/1 -> mux/2
  DCM31/1 -> mux/3
  [u3] -> DCM12/1
  [u5] -> DCM12/2
  [u3] -> P5/1
  [u2] -> P5/2
  [u1] -> P5/3
  [u6] -> P7/1
  [u4] -> P7/2
  P5/1 -> DCM22/1
  P7/1 -> DCM22/2
  DCM22/1 -> mux/5
  [u3] -> P6/1
  [u2] -> P6/2
  [u4] -> P6/3
  [u6] -> P8/1
  [u1] -> P8/2
  P6/1 -> DCM32/1
  P8/1 -> DCM32/2
  DCM32/1 -> mux/6
  [u6] -> DCM11/1
  [u5] -> DCM11/2
  DCM11/1 -> mux/1
  [u2] -> DCM13/1
  DCM13/1 -> mux/7
  [u1] -> DCM23/2
  [u5] -> DCM23/1
  DCM23/1 -> mux/8
  [u4] -> DCM33/2
  [u5] -> DCM33/1
  DCM33/1 -> mux/9

== system SimpleEKF_2007a/INS/Attitude update/Stage2/eulerToQuat ==
  attInitCon : Inport  OutDataType=fixdt(1,16,0)  OutScaling=[]
  Mux : Mux
  a1 : Subsystem
  a2 : Subsystem
  a3 : Subsystem
  a4 : Subsystem
  q : Outport  OutDataType=fixdt(1,16,0)  OutScaling=[]
  wires:
  a1/1(a1) -> Mux/1
  a2/1(a2) -> Mux/2
  a3/1(a3) -> Mux/3
  a4/1(a2) -> Mux/4
  Mux/1 -> q/1
  attInitCon/1 -> a1/1(attInitCon), a3/1(attInitCon), a4/1(attInitCon), a2/1(attInitCon)

== system SimpleEKF_2007a/INS/Attitude update/Stage2/square ==
  squareLibIn : Inport  DataType=double  OutDataType=fixdt(1,16,0)  OutScaling=[]
  Product : Product  OutDataType=fixdt(1,16,0)  OutScaling=[]  RndMeth=Zero
  squareLibOut : Outport  OutDataType=fixdt(1,16,0)  OutScaling=[]  InitialOutput=0
  wires:
  squareLibIn/1 -> Product/2, Product/1
  Product/1 -> squareLibOut/1

== system SimpleEKF_2007a/INS/Attitude update/Stage2/square1 ==
  squareLibIn : Inport  DataType=double  OutDataType=fixdt(1,16,0)  OutScaling=[]
  Product : Product  OutDataType=fixdt(1,16,0)  OutScaling=[]  RndMeth=Zero
  squareLibOut : Outport  OutDataType=fixdt(1,16,0)  OutScaling=[]  InitialOutput=0
  wires:
  squareLibIn/1 -> Product/2, Product/1
  Product/1 -> squareLibOut/1

== system SimpleEKF_2007a/INS/Attitude update/Stage2/square2 ==
  squareLibIn : Inport  DataType=double  OutDataType=fixdt(1,16,0)  OutScaling=[]
  Product : Product  OutDataType=fixdt(1,16,0)  OutScaling=[]  RndMeth=Zero
  squareLibOut : Outport  OutDataType=fixdt(1,16,0)  OutScaling=[]  InitialOutput=0
  wires:
  squareLibIn/1 -> Product/2, Product/1
  Product/1 -> squareLibOut/1

== system SimpleEKF_2007a/INS/Coriolis correction/RM/square ==
  squareLibIn : Inport  DataType=double  OutDataType=fixdt(1,16,0)  OutScaling=[]
  Product : Product  OutDataType=fixdt(1,16,0)  OutScaling=[]  RndMeth=Zero
  squareLibOut : Outport  OutDataType=fixdt(1,16,0)  OutScaling=[]  InitialOutput=0
  wires:
  squareLibIn/1 -> Product/2, Product/1
  Product/1 -> squareLibOut/1

== system SimpleEKF_2007a/INS/Coriolis correction/RM/square1 ==
  squareLibIn : Inport  DataType=double  OutDataType=fixdt(1,16,0)  OutScaling=[]
  Product : Product  OutDataType=fixdt(1,16,0)  OutScaling=[]  RndMeth=Zero
  squareLibOut : Outport  OutDataType=fixdt(1,16,0)  OutScaling=[]  InitialOutput=0
  wires:
  squareLibIn/1 -> Product/2, Product/1
  Product/1 -> squareLibOut/1

== system SimpleEKF_2007a/INS/Coriolis correction/RN/square ==
  squareLibIn : Inport  DataType=double  OutDataType=fixdt(1,16,0)  OutScaling=[]
  Product : Product  OutDataType=fixdt(1,16,0)  OutScaling=[]  RndMeth=Zero
  squareLibOut : Outport  OutDataType=fixdt(1,16,0)  OutScaling=[]  InitialOutput=0
  wires:
  squareLibIn/1 -> Product/2, Product/1
  Product/1 -> squareLibOut/1

== system SimpleEKF_2007a/INS/Coriolis correction/RN/square1 ==
  squareLibIn : Inport  DataType=double  OutDataType=fixdt(1,16,0)  OutScaling=[]
  Product : Product  OutDataType=fixdt(1,16,0)  OutScaling=[]  RndMeth=Zero
  squareLibOut : Outport  OutDataType=fixdt(1,16,0)  OutScaling=[]  InitialOutput=0
  wires:
  squareLibIn/1 -> Product/2, Product/1
  Product/1 -> squareLibOut/1

== system SimpleEKF_2007a/Trajectory  Generator/Signals Conversions dtgen/Subsystem1/square ==
  squareLibIn : Inport  DataType=double  OutDataType=fixdt(1,16,0)  OutScaling=[]
  Product : Product  OutDataType=fixdt(1,16,0)  OutScaling=[]  RndMeth=Zero
  squareLibOut : Outport  OutDataType=fixdt(1,16,0)  OutScaling=[]  InitialOutput=0
  wires:
  squareLibIn/1 -> Product/2, Product/1
  Product/1 -> squareLibOut/1

== system SimpleEKF_2007a/EKF/MeasureVector/GPS/Subsystem1/square ==
  squareLibIn : Inport  DataType=double  OutDataType=fixdt(1,16,0)  OutScaling=[]
  Product : Product  OutDataType=fixdt(1,16,0)  OutScaling=[]  RndMeth=Zero
  squareLibOut : Outport  OutDataType=fixdt(1,16,0)  OutScaling=[]  InitialOutput=0
  wires:
  squareLibIn/1 -> Product/2, Product/1
  Product/1 -> squareLibOut/1

== system SimpleEKF_2007a/EKF/MeasureVector/GPS/Subsystem2/square ==
  squareLibIn : Inport  DataType=double  OutDataType=fixdt(1,16,0)  OutScaling=[]
  Product : Product  OutDataType=fixdt(1,16,0)  OutScaling=[]  RndMeth=Zero
  squareLibOut : Outport  OutDataType=fixdt(1,16,0)  OutScaling=[]  InitialOutput=0
  wires:
  squareLibIn/1 -> Product/2, Product/1
  Product/1 -> squareLibOut/1

== system SimpleEKF_2007a/INS/Attitude update/Stage1/Subsystem/Subsystem ==
  M11 : Inport  OutDataType=fixdt(1,16,0)  OutScaling=[]
  M21 : Inport  Port=2  OutDataType=fixdt(1,16,0)  OutScaling=[]
  M31 : Inport  Port=3  OutDataType=fixdt(1,16,0)  OutScaling=[]
  M12 : Inport  Port=4  OutDataType=fixdt(1,16,0)  OutScaling=[]
  M22 : Inport  Port=5  OutDataType=fixdt(1,16,0)  OutScaling=[]
  M32 : Inport  Port=6  OutDataType=fixdt(1,16,0)  OutScaling=[]
  M13 : Inport  Port=7  OutDataType=fixdt(1,16,0)  OutScaling=[]
  M23 : Inport  Port=8  OutDataType=fixdt(1,16,0)  OutScaling=[]
  M33 : Inport  Port=9  OutDataType=fixdt(1,16,0)  OutScaling=[]
  Mux : Mux  Inputs=9
  Reshape (9) to [3x3] column-major : Reshape  OutputDimensionality=Customize  OutputDimensions=[3,3]
  Matrix : Outport  OutDataType=fixdt(1,16,0)  OutScaling=[]
  wires:
  M33/1 -> Mux/9
  M23/1 -> Mux/8
  M13/1 -> Mux/7
  M32/1 -> Mux/6
  Reshape (9) to [3x3] column-major/1 -> Matrix/1
  M22/1 -> Mux/5
  M12/1 -> Mux/4
  M31/1 -> Mux/3
  M21/1 -> Mux/2
  M11/1 -> Mux/1
  Mux/1 -> Reshape (9) to [3x3] column-major/1

== system SimpleEKF_2007a/INS/Attitude update/Stage1/Subsystem/a11 ==
  quat : Inport  OutDataType=fixdt(1,16,0)  OutScaling=[]  Interpolate=off  mask(Inport (HW)){maskPort=1, PortWidth=0, BusOuputAsStruct=0, signalName=<, Unit=, lowerRange=, upperRange=, InitOut=, latch=Latched}
      mask prompts: maskPort "Mask Port"; PortWidth "Dimensions (-1 for dynamic):"; BusOuputAsStruct "Output as Non-Virtual:"; signalName "Signal Name"; lowerRange "Lower Range"; upperRange "Upper Range"; InitOut "Software Initial Output"; latch "DEOS Consumed Type"
      mask init:
      | %hwbcalib_inport(gcbh,'done');
      settings: CopyFcn=hwbcalib_copyfcn(gcbh);  UndoDeleteFcn=hwbcalib_inport(gcbh,'undodelete');  ModelCloseFcn=set_param(gcbh,'DeleteFcn','');  OpenFcn=hwbcalib_inport(gcbh,0);  PreDeleteFcn=hwbcalib_inport(gcbh,'delete');
      mask Help: file:///../../../Inport.html
      mask StyleString: edit,edit,edit,edit,edit,edit,edit,edit,popup(Latched|Not Latched)
      mask Display:
      | text(4,8,['quat   [' maskPort ']'],'Horizontal','left','Vertical','middle')
      | plot([0 50-10],[0 0]);
      | plot([0 0],[0 16]);
      | plot([0 50-10],[16 16]);
      | plot([50-10 50],[16 8]);
      | plot([50-10 50],[0 8]);
  BorderBottom : Subsystem
      settings: AttributesFormatString="* HONEYWELL PROPRIETARY AND CONFIDENTIAL * Copyright (c) 1996-2011 Honeywell International Inc. * Unpublished Work.  All rights reserved. *"
      mask Type: Border (HW)
      mask Description: Border
  BorderLeft : Subsystem
      mask Type: Border (HW)
      mask Description: Border
  BorderRight : Subsystem
      mask Type: Border (HW)
      mask Description: Border
  BorderTop : Subsystem
      mask Type: Border (HW)
      mask Description: Border
  Subsystem Revision : Subsystem  mask(Subsystem Revision (HW)){trace=}
      mask prompts: trace "Trace Tag:"
      settings: CopyFcn=hwbcalib_copyfcn(gcbh);  OpenFcn=hwbcalib_subrevision(gcbh,0);
      mask Help: file:///../../../Subsystem_Revision.html
      mask Display: disp('Program: \nCPU/Process: /D:\nDLL: tgen\nFilename: INS_ham_napokusy.mdl\nSubsystem: INS/Attitude update/Stage1/quatToDcm/a11\n\nHAM Library Version: 6.5.0\nRevision: -\nDate: 07-Dec-2011 at 09:52:57\nModel Update Rate: 100 Hz\n[ode3]\nTrace Tag: \n\nPage: 13 of 53, Parent Page: 12')
  deMux : Subsystem  mask(Demux (HW)){num=4}
      mask prompts: num "Number of Outputs"
      mask init:
      | %hwbcalib_doDoneCallback('hwbcalib_demux',gcbh,99);
      settings: CopyFcn=hwbcalib_copyfcn(gcbh);  OpenFcn=hwbcalib_demux(gcbh,0);
      mask Help: file:///../../../De-Multiplexer.html
  product : Subsystem  mask(Product (HW)){num=2}
      mask prompts: num "Numer of Inputs"
      mask init:
      | %hwbcalib_doDoneCallback('hwbcalib_product',gcbh,99);
      settings: CopyFcn=hwbcalib_copyfcn(gcbh);  OpenFcn=hwbcalib_product(gcbh,0);
      mask Help: file:///../../../Product.html
      mask Display: disp('X')
  product1 : Subsystem  mask(Product (HW)){num=2}
      mask prompts: num "Numer of Inputs"
      mask init:
      | %hwbcalib_doDoneCallback('hwbcalib_product',gcbh,99);
      settings: CopyFcn=hwbcalib_copyfcn(gcbh);  OpenFcn=hwbcalib_product(gcbh,0);
      mask Help: file:///../../../Product.html
      mask Display: disp('X')
  product2 : Subsystem  mask(Product (HW)){num=2}
      mask prompts: num "Numer of Inputs"
      mask init:
      | %hwbcalib_doDoneCallback('hwbcalib_product',gcbh,99);
      settings: CopyFcn=hwbcalib_copyfcn(gcbh);  OpenFcn=hwbcalib_product(gcbh,0);
      mask Help: file:///../../../Product.html
      mask Display: disp('X')
  product3 : Subsystem  mask(Product (HW)){num=2}
      mask prompts: num "Numer of Inputs"
      mask init:
      | %hwbcalib_doDoneCallback('hwbcalib_product',gcbh,99);
      settings: CopyFcn=hwbcalib_copyfcn(gcbh);  OpenFcn=hwbcalib_product(gcbh,0);
      mask Help: file:///../../../Product.html
      mask Display: disp('X')
  sum : Subsystem  mask(Sum (HW)){signs=++--}
      mask prompts: signs "String of Signs"
      mask init:
      | %hwbcalib_doDoneCallback('hwbcalib_sum',gcbh,99);
      settings: CopyFcn=hwbcalib_copyfcn(gcbh);  OpenFcn=hwbcalib_sum(gcbh,0);
      mask Help: file:///../../../Summation.html
      mask Display:
      | text(0.2, (20*(4-1)+11)/80, '+');
      | text(0.2, (20*(3-1)+11)/80, '+');
      | text(0.2, (20*(2-1)+11)/80, '-');
      | text(0.2, (20*(1-1)+11)/80, '-');
  a11 : Outport  OutDataType=fixdt(1,16,0)  OutScaling=[]  mask(Outport (HW)){maskPort=1, PortWidth=0, lowerRange=, upperRange=, signalName=<, Unit=}
      mask prompts: maskPort "Mask Port"; PortWidth "Dimensions (-1 for dynamic):"; lowerRange "Lower Range"; upperRange "Upper Range"; signalName "Signal Name"; Unit "Units"
      mask init:
      | %hwbcalib_outport(gcbh,'done');
      settings: CopyFcn=hwbcalib_copyfcn(gcbh);  UndoDeleteFcn=hwbcalib_outport(gcbh,'undodelete');  ModelCloseFcn=set_param(gcbh,'DeleteFcn','');  OpenFcn=hwbcalib_outport(gcbh,0);  PreDeleteFcn=hwbcalib_outport(gcbh,'delete');
      mask Help: file:///../../../Outport.html
      mask Display:
      | text(50-4,8,['a11   [' maskPort ']'],'Horizontal','right','Vertical','middle')
      | plot([10 50],[0 0]);
      | plot([50-1 50-1],[0 16]);
      | plot([10 50],[16 16]);
      | plot([0 10],[8 16]);
      | plot([0 10],[8 0]);
  wires:
  quat/1 -> deMux/1(Dmx)
  sum/1(1000) -> a11/1
  deMux/1(1) -> product/2(2), product/1(1)
  deMux/2(2) -> product1/1(1), product1/2(2)
  deMux/3(3) -> product2/1(1), product2/2(2)
  deMux/4(4) -> product3/2(2), product3/1(1)
  product/1(1000) -> sum/1(1)
  product1/1(1000) -> sum/2(2)
  product2/1(1000) -> sum/3(3)
  product3/1(1000) -> sum/4(4)
